simulink model "CupeledPendelums_simple_D_K"  (R2013a)
settings: Solver=ode4  StartTime=0.0  StopTime=5.0  FixedStep=0.001  RelTol=1e-3
undefined symbols (not defined in the file): alpha, D, K, psi1_0, psi1_dot_0, psi2_0, psi2_dot_0
settings Model: Creator=USER  LastModifiedBy=USER

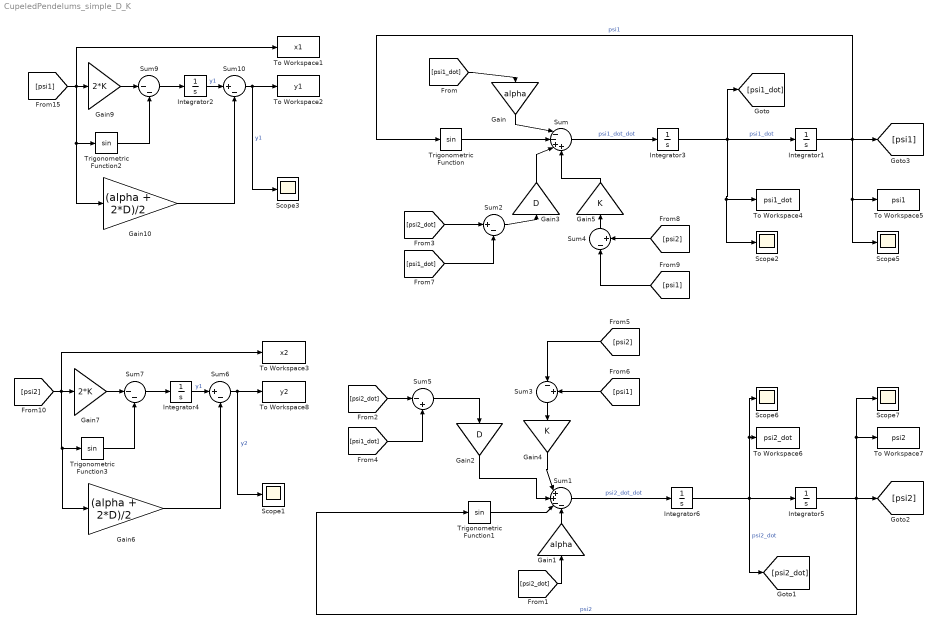
== system CupeledPendelums_simple_D_K ==
  Gain : Gain  Gain=alpha
  Gain1 : Gain  Gain=alpha
  Gain10 : Gain  Gain=(alpha + 2*D)/2
  Gain2 : Gain  Gain=D
  Gain3 : Gain  Gain=D
  Gain4 : Gain  Gain=K
  Gain5 : Gain  Gain=K
  Gain6 : Gain  Gain=(alpha + 2*D)/2
  Gain7 : Gain  Gain=2*K
  Gain9 : Gain  Gain=2*K
  Integrator1 : Integrator  InitialCondition=psi1_0
  Integrator2 : Integrator  InitialCondition=(alpha+2*D)*psi1_0+psi1_dot_0
  Integrator3 : Integrator  InitialCondition=psi1_dot_0
  Integrator4 : Integrator  InitialCondition=(alpha+2*D)*psi2_0+psi2_dot_0
  Integrator5 : Integrator  InitialCondition=psi2_0
  Integrator6 : Integrator  InitialCondition=psi2_dot_0
  Scope{1..3,5..7} (6 alike) : Scope
      Scope2 settings: SaveName=ScopeData2
      Scope5 settings: SaveName=ScopeData5
      Scope6 settings: SaveName=ScopeData6
      Scope7 settings: SaveName=ScopeData7
  Sum : Sum  Inputs=|--++
  Sum1 : Sum  Inputs=|++--
  Sum10 : Sum  Inputs=|+-
  Sum2 : Sum  Inputs=|+-
  Sum3 : Sum  Inputs=|-+
  Sum4 : Sum  Inputs=|-+
  Sum5 : Sum  Inputs=|-+
  Sum6 : Sum  Inputs=|+-
  Sum7 : Sum  Inputs=|--
  Sum9 : Sum  Inputs=|--
  To Workspace1 : ToWorkspace  VariableName=x1  SampleTime=-1  SaveFormat=Timeseries
  To Workspace2 : ToWorkspace  VariableName=y1  SampleTime=-1  SaveFormat=Timeseries
  To Workspace3 : ToWorkspace  VariableName=x2  SampleTime=-1  SaveFormat=Timeseries
  To Workspace4 : ToWorkspace  VariableName=psi1_dot  SampleTime=-1  SaveFormat=Timeseries
  To Workspace5 : ToWorkspace  VariableName=psi1  SampleTime=-1  SaveFormat=Timeseries
  To Workspace6 : ToWorkspace  VariableName=psi2_dot  SampleTime=-1  SaveFormat=Timeseries
  To Workspace7 : ToWorkspace  VariableName=psi2  SampleTime=-1  SaveFormat=Timeseries
  To Workspace8 : ToWorkspace  VariableName=y2  SampleTime=-1  SaveFormat=Timeseries
  Trigonometric Function{,1..3} (4 alike) : Trigonometry
  wires:
  Sum/1 -> Integrator3/1  "psi1_dot_dot"
  Integrator3/1 -> Scope2/1, To Workspace4/1, [psi1_dot], Integrator1/1  "psi1_dot"
  [psi1_dot] -> Gain/1
  Gain/1 -> Sum/1
  Trigonometric Function/1 -> Sum/2
  Sum2/1 -> Gain3/1
  [psi2_dot] -> Sum2/1
  [psi1_dot] -> Sum2/2
  Sum1/1 -> Integrator6/1  "psi2_dot_dot"
  [psi2_dot] -> Gain1/1
  Sum5/1 -> Gain2/1
  [psi2_dot] -> Sum5/1
  [psi1_dot] -> Sum5/2
  Gain2/1 -> Sum1/2
  Gain1/1 -> Sum1/4
  Integrator1/1 -> [psi1], Trigonometric Function/1, Scope5/1, To Workspace5/1  "psi1"
  Integrator6/1 -> Scope6/1, To Workspace6/1, [psi2_dot], Integrator5/1  "psi2_dot"
  Integrator5/1 -> Trigonometric Function1/1, [psi2], To Workspace7/1, Scope7/1  "psi2"
  Sum3/1 -> Gain4/1
  Gain4/1 -> Sum1/1
  [psi2] -> Sum3/1
  [psi1] -> Sum3/2
  Gain5/1 -> Sum/4
  Sum4/1 -> Gain5/1
  [psi1] -> Sum4/1
  [psi2] -> Sum4/2
  Gain3/1 -> Sum/3
  Trigonometric Function1/1 -> Sum1/3
  Sum10/1 -> Scope3/1, To Workspace2/1  "y1"
  Sum9/1 -> Integrator2/1
  Gain9/1 -> Sum9/1
  [psi1] -> To Workspace1/1, Gain10/1, Trigonometric Function2/1, Gain9/1
  Trigonometric Function2/1 -> Sum9/2
  Integrator2/1 -> Sum10/1  "y1"
  Gain10/1 -> Sum10/2
  Sum6/1 -> Scope1/1, To Workspace8/1  "y2"
  Sum7/1 -> Integrator4/1
  Gain7/1 -> Sum7/1
  [psi2] -> To Workspace3/1, Gain6/1, Trigonometric Function3/1, Gain7/1
  Trigonometric Function3/1 -> Sum7/2
  Integrator4/1 -> Sum6/1  "y1"
  Gain6/1 -> Sum6/2
